simulink model "DEM_testbench"  (Simulink 7.9)
settings: Solver=FixedStepDiscrete  StartTime=0.0  StopTime=simu.trantime  RelTol=1e-3
undefined symbols (not defined in the file): dac, Fs
libraries: dspsrcs4 x2
settings Model: Creator=amyles  LastModifiedBy=Arnaldi Isacco
settings DataIOCC: MaxDataPoints=50000
settings DebuggingCC: ParameterPrecisionLossMsg=none  StrictBusMsg=Warning
settings SFSimCC: SimParseCustomCode=off
settings CodeAppCC: CustomSymbolStrType=$N$R$M_T
settings GRTTargetCC: CombineOutputUpdateFcns=off  GRTInterface=on

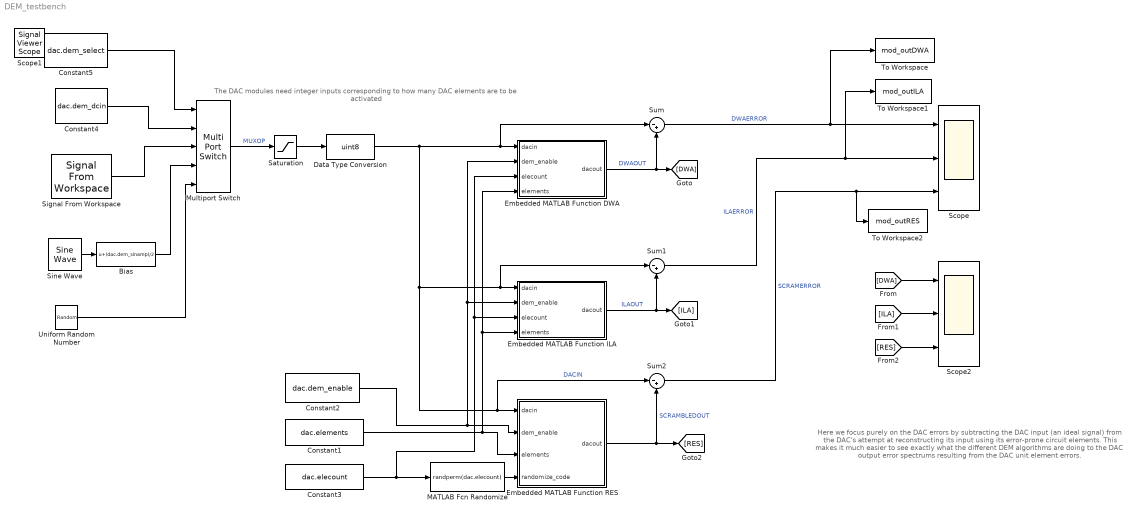
== system DEM_testbench ==
  note: The DAC modules need integer
      | inputs corresponding to how many
      | DAC elements are to be activated
  note: Here we focus purely on the DAC errors by
      | subtracting the DAC input (an ideal signal) from the
      | DAC's attempt at reconstructing its input using its
      | error-prone circuit elements.
      |
      | This makes it much easier to see exactly what the different
      | DEM algorithms are doing to the DAC output error
      | spectrums resulting from the DAC unit element errors.
  Bias : Bias  Bias=(dac.dem_sinamp)/2
  Constant1 : Constant  Value=dac.elements  SampleTime=1/Fs
  Constant2 : Constant  Value=dac.dem_enable  SampleTime=1/Fs
  Constant3 : Constant  Value=dac.elecount  SampleTime=1/Fs
  Constant4 : Constant  Value=dac.dem_dcin  SampleTime=1/Fs
  Constant5 : Constant  Value=dac.dem_select  SampleTime=1/Fs
  Data Type Conversion : DataTypeConversion  OutDataTypeStr=uint8  RndMeth=Nearest
  Embedded MATLAB Function DWA : MATLAB Function  TreatAsAtomicUnit=on
  Embedded MATLAB Function ILA : MATLAB Function  TreatAsAtomicUnit=on
  Embedded MATLAB Function RES : MATLAB Function  TreatAsAtomicUnit=on
  MATLAB Fcn Randomize : MATLABFcn  MATLABFcn=randperm(dac.elecount)  SampleTime=1/Fs
  Multiport Switch : MultiPortSwitch  Inputs=4  zeroidx=off  SampleTime=1/Fs
  Saturation : Saturate  UpperLimit=dac.elecount  LowerLimit=0  SampleTime=1/Fs
  Scope : Scope  NumInputPorts=3
      settings: TimeRange=0.0018  YMin=-0.04~-5~-0.06  YMax=0.04~5~0.06
  Scope2 : Scope  NumInputPorts=3
      settings: TimeRange=0.0006018447348193692  YMin=1.96~1.94~1.94  YMax=2.06~2.06~2.06
  Signal From Workspace : dspsrcs4/Signal From Workspace  X=[1 1 2]  Ts=1/Fs  nsamps=1  OutputAfterFinalValue=Cyclic repetition  ignoreOrWarnInputAndFrameLengths=off
  Sine Wave : dspsrcs4/Sine Wave  Amplitude=(dac.dem_sinamp)/2  Frequency=dac.dem_sinfreq  Phase=0  SampleMode=Discrete  OutComplex=Real  CompMethod=Trigonometric fcn  TableSize=Speed  SampleTime=1/Fs  SamplesPerFrame=1  ResetState=Restart at time zero  dataType=double  wordLen=16  udDataType=sfix(16)  fracBitsMode=Best precision  numFracBits=15  OutDataTypeStr=double  LastOutDataTypeStr=double
  Sum : Sum  Inputs=|-+  SampleTime=1/Fs
  Sum1 : Sum  Inputs=|-+  SampleTime=1/Fs
  Sum2 : Sum  Inputs=|-+  SampleTime=1/Fs
  To Workspace : ToWorkspace  VariableName=mod_outDWA  SampleTime=-1
  To Workspace1 : ToWorkspace  VariableName=mod_outILA  SampleTime=-1
  To Workspace2 : ToWorkspace  VariableName=mod_outRES  SampleTime=-1
  Uniform Random Number : UniformRandomNumber  Minimum=0  Maximum=dac.elecount  SampleTime=1/Fs
  Scope1 : SignalViewerScope  IOType=viewer  NumInputPorts=5  ZoomMode=xonly  RefreshTime=0.035000
      settings: YMin=0~0~-5~-5~-5  YMax=3~3~5~5~5
  wires:
  Constant5/1 -> Multiport Switch/1
  Signal From Workspace/1 -> Multiport Switch/3
  Sine Wave/1 -> Bias/1
  Multiport Switch/1 -> Saturation/1  "MUXOP"
  Data Type Conversion/1 -> Embedded MATLAB Function DWA/1(dacin), Sum/1, Embedded MATLAB Function ILA/1(dacin), Sum1/1, Sum2/1, Embedded MATLAB Function RES/1(dacin)  "DACIN"
  Saturation/1 -> Data Type Conversion/1
  Bias/1 -> Multiport Switch/4
  Uniform Random Number/1 -> Multiport Switch/5
  Constant4/1 -> Multiport Switch/2
  Embedded MATLAB Function DWA/1(dacout) -> Sum/2, [DWA]  "DWAOUT"
  Embedded MATLAB Function ILA/1(dacout) -> Sum1/2, [ILA]  "ILAOUT"
  Embedded MATLAB Function RES/1(dacout) -> Sum2/2, [RES]  "SCRAMBLEDOUT"
  Sum/1 -> Scope/1, To Workspace/1  "DWAERROR"
  Sum1/1 -> Scope/2, To Workspace1/1  "ILAERROR"
  Sum2/1 -> Scope/3, To Workspace2/1  "SCRAMERROR"
  Constant3/1 -> MATLAB Fcn Randomize/1, Embedded MATLAB Function ILA/3(elecount), Embedded MATLAB Function DWA/3(elecount)
  MATLAB Fcn Randomize/1 -> Embedded MATLAB Function RES/4(randomize_code)
  Constant2/1 -> Embedded MATLAB Function DWA/2(dem_enable), Embedded MATLAB Function ILA/2(dem_enable), Embedded MATLAB Function RES/2(dem_enable)
  Constant1/1 -> Embedded MATLAB Function ILA/4(elements), Embedded MATLAB Function DWA/4(elements), Embedded MATLAB Function RES/3(elements)
  [DWA] -> Scope2/1
  [ILA] -> Scope2/2
  [RES] -> Scope2/3

== matlab function Embedded MATLAB Function ILA ==
  data: dacin input double; dacout output double; dem_enable input double; elecount input double; elements input double
function dacout = DAC(dacin, dem_enable, elecount, elements)
%% ------------------ INDIVIDUAL LEVEL AVERAGING DEM ----------------------
%
% This function performs ILA DEM and assumes the routines load_par has been
% compiled in order to load the dac structure needed for the code to function.

%% FUNCTION CODE:

persistent ila_pointer; % Persistent rotator state

dacplus1 = dacin+1; % Quantizer starts at 0, MATLAB array indices at 1...
                    
% DEM DISABLED:

if isempty(ila_pointer) || (dem_enable == 0)
    ila_pointer = ones(1,32);    % Initialize indices and reset if not rotating.
                                 % Assume a max of 32 DAC elements (5 Bit)
end

% DEM ENABLED:

dacout = 0.0;
point = ila_pointer(1,dacplus1);

for indx = 1:1:dacin
    dacout = dacout + elements(point);
    point = mod(point, elecount) + 1;
end

ila_pointer(1,dacplus1) = point;

end

== matlab function Embedded MATLAB Function DWA ==
  data: dacin input double; dacout output double; dem_enable input double; elecount input double; elements input double
function dacout = DAC(dacin, dem_enable, elecount, elements)
%% ------------------- DATA WEIGHTING AVERAGING DEM -----------------------
%
% This function performs DWA DEM and assumes the routines load_par has been
% compiled in order to load the dac structure needed for the code to function.

%% FUNCTION CODE:

persistent dwa_pointer; % Persistent rotator state

% DEM DISABLED:

if isempty(dwa_pointer) || (dem_enable == 0)
    dwa_pointer = 1;    % Reset if not rotating
end

% DEM ENABLED:

dacout = 0.0;

for indx = 1:1:dacin
    dacout = dacout + elements(dwa_pointer);
    dwa_pointer = dwa_pointer + 1;
    if (dwa_pointer > elecount)
        dwa_pointer = 1;
    end
end

end

== matlab function Embedded MATLAB Function RES ==
  data: dacin input double; dacout output double; dem_enable input double; elements input double; randomize_code input double
function dacout = DAC(dacin, dem_enable, elements, randomize_code)
%% ------------------- RANDOM ELEMENT SELECTION DEM -----------------------

% The Random Element Selection DEM code is used to lineatize the DAC in a
% time average fashion. However it turns the mismatch errors into a white
% noise, some of which will affect the signal band of interest.
%
% This function assumes the routines load_par has been compiled in order to
% load the dac structure needed for the code to function.
%
% The function allows dynamic resizing of the DAC by using the actual
% randomization code from an external function.

%% FUNCTION CODE:

if (dem_enable == 0)
    dacout = sum(elements(1:dacin));
else
    dacout = sum(elements(randomize_code(1:dacin)));
end

end
